simulink model "test_simu"  (R2016a)
settings: Solver=VariableStepAuto  StartTime=0.0  StopTime=10.0  RelTol=1e-3
values from neighbouring files (symbols this model uses):
  g = 9.81    [controller_script.m]
  I = [0.06 0.003 0.0006;0.003 0.05 0.002;0.002 0.003 0.1]    [controller_script.m]
  m = 1.5    [controller_script.m]
settings Model: Creator=hugoa  LastModifiedBy=ALEX

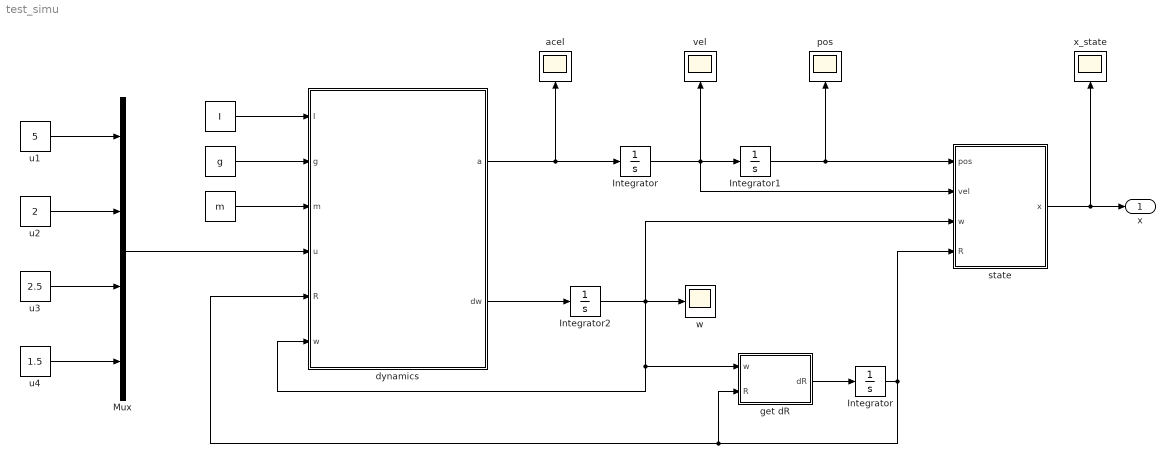
== system test_simu ==
  " " : Constant  Value=I
  "  " : Constant  Value=g
  "   " : Constant  Value=m
  " u1 " : Constant  Value=5
  " u2" : Constant  Value=2
  " u3" : Constant  Value=2.5
  " u4" : Constant  Value=1.5
  Integrator : Integrator  InitialCondition=[0;0;0]
  "Integrator " : Integrator  InitialCondition=eye(3)  LimitOutput=on  UpperSaturationLimit=1  LowerSaturationLimit=0
  Integrator1 : Integrator  InitialCondition=[0;0;0]
  Integrator2 : Integrator  InitialCondition=[0;0;0]
  Mux : Mux
  acel : Scope
  dynamics : MATLAB Function  TreatAsAtomicUnit=on
  get dR : MATLAB Function  TreatAsAtomicUnit=on
  pos : Scope
  state : MATLAB Function  TreatAsAtomicUnit=on
  vel : Scope
  w : Scope
  x_state : Scope
  x : Outport
  wires:
  dynamics/2(dw) -> Integrator2/1
  get dR/1(dR) -> "Integrator "/1
  "Integrator "/1 -> state/4(R), dynamics/5(R), get dR/2(R)
  Mux/1 -> dynamics/4(u)
  " u1 "/1 -> Mux/1
  " u2"/1 -> Mux/2
  " u3"/1 -> Mux/3
  " u4"/1 -> Mux/4
  dynamics/1(a) -> acel/1, Integrator/1
  Integrator2/1 -> state/3(w), w/1, dynamics/6(w), get dR/1(w)
  Integrator/1 -> vel/1, Integrator1/1, state/2(vel)
  Integrator1/1 -> pos/1, state/1(pos)
  state/1(x) -> x_state/1, x/1
  " "/1 -> dynamics/1(I)
  "   "/1 -> dynamics/3(m)
  "  "/1 -> dynamics/2(g)

== matlab function test_simu/get dR ==
  data: w input; dR output; R input
function dR = fcn(w, R)
%#codegen
r = 1; p = 3; q =2;
skew_w = [0,-w(3),w(2); w(3),0,-w(1); -w(2),w(1),0];



dR = R*skew_w;

== matlab function test_simu/dynamics ==
  data: I input; g input; m input; u input; R input; a output; w input size=3; dw output
function [a,dw] = fcn(I,g,m,u,R,w)
%#codegen

% VARIÁVEIS

%m = 1;                          %mass of drone
%I = [0.06 0.003 0.0006;0.001 0.05 0.002; 0.002 0.003 0.1];        %inertial matrix 
%g = 9.81;                       %gravitational force
zw = [0;0;1];
zB = R*zw;

r = 1; p = 3; q =2;
skew_w = [0,-w(3),w(2); w(3),0,-w(1); -w(2),w(1),0];
uT = [u(2);u(3);u(4)];



a = -g*zw+(u(1)/m)*zB;
dw = inv(I)*(-skew_w*I*w + uT);

%FALTA UT - NOT WORKING
%dw = inv(I)*(-skew_w*I*w + uT);

== matlab function test_simu/state ==
  data: pos input; vel input; w input; R input; x output
function x = fcn(pos, vel, w, R)
%#codegen
R_euler = transpose(rotm2eul(R));

x = [pos, vel, w, R_euler];
